simulink model "conversions_bad"  (R2026a)
settings: Solver=VariableStepAuto  StopTime=267365
undefined symbols (not defined in the file or in its folder): IAU
libraries: aerolibtransform2 x1
settings Model: Creator=syane  LastModifiedBy=syane

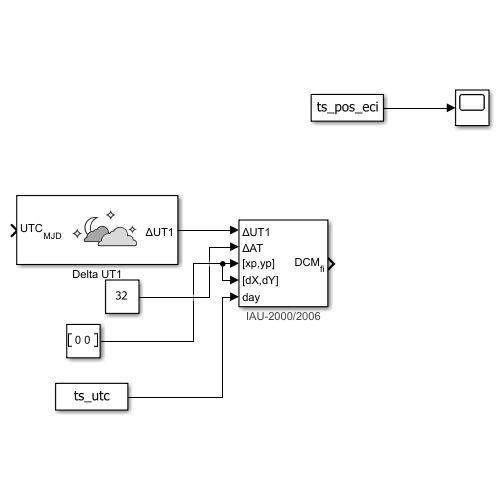
[thumbnail: Simulink's stored preview of the top-level diagram]
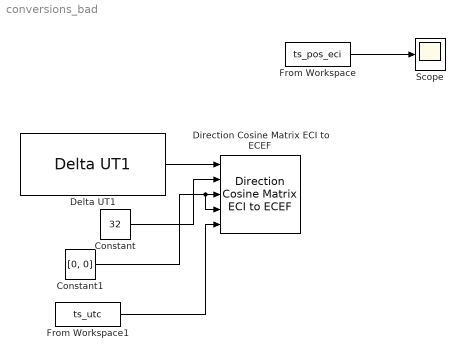
== system conversions_bad ==
  Constant : Constant  Value=32
  Constant1 : Constant  Value=[0, 0]
  Delta UT1 : DeltaUT1
  Direction Cosine Matrix ECI to ECEF : aerolibtransform2/Direction Cosine Matrix ECI to ECEF  red=IAU-2000/2006  year=2013  month=January  day=1  hour=0  min=0  sec=0  deltaT=Day  errorflag=Error  extraparamflag=on
      settings: AttributesFormatString=%<red>
  From Workspace : FromWorkspace  VariableName=ts_pos_eci
  From Workspace1 : FromWorkspace  VariableName=ts_utc
  Scope : Scope
      settings: ActiveDisplayYMinimum=-5.3051903863951579E+7  ActiveDisplayYMaximum=5.3259075173262589E+7
  wires:
  From Workspace/1 -> Scope/1
  Delta UT1/1 -> Direction Cosine Matrix ECI to ECEF/1
  Constant/1 -> Direction Cosine Matrix ECI to ECEF/2
  Constant1/1 -> Direction Cosine Matrix ECI to ECEF/4, Direction Cosine Matrix ECI to ECEF/3
  From Workspace1/1 -> Direction Cosine Matrix ECI to ECEF/5
